simulink model "prob1"  (R2020b)
settings: Solver=VariableStepAuto  StartTime=0.0  StopTime=10.0  RelTol=1e-3
settings Model: Creator=nadee  LastModifiedBy=nadee

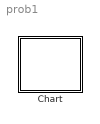
== system prob1 ==
  Chart : Stateflow chart  TreatAsAtomicUnit=on

== stateflow chart prob1/Chart ==
